simulink model "image_crop"  (R2016a)
settings: Solver=VariableStepAuto  StartTime=0.0  StopTime=1  RelTol=1e-3
libraries: visionsources x1
settings Model: Creator=Yewly  LastModifiedBy=Yewly

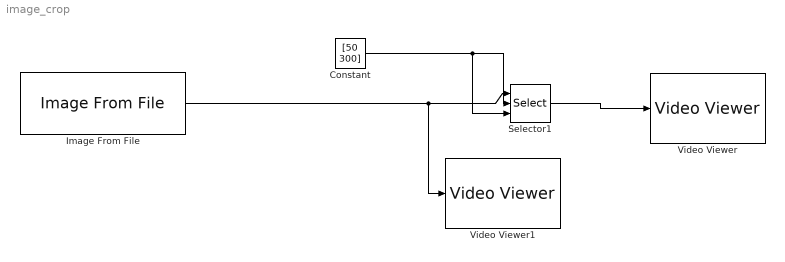
== system image_crop ==
  Constant : Constant  Value=[50 300]
  Image From File : visionsources/Image From File  Tag=vipblks_nd  FileName=color6.jpg  imagePorts=One multidimensional signal  Ts=1  ImageDataType=Inherit from input image  Signed=on  WordLength=16  sdImageDataType=uint(8)  FractionLengthMode=User-defined  FractionLength=15  OutPortLabels=R|G|B
  Selector1 : Selector  NumberOfDimensions=3  InputPortWidth=2  IndexOptions=Starting and ending indices (port),Starting and ending indices (port),Starting index (dialog)  Indices=50,50,1  OutputSizes=300,300,3
  Video Viewer : VideoViewer  FigPos=[886.6 726.8 540 585.6]
  Video Viewer1 : VideoViewer  FigPos=[285.8 732.4 540 585.6]
  wires:
  Selector1/1 -> Video Viewer/1
  Image From File/1 -> Selector1/1, Video Viewer1/1
  Constant/1 -> Selector1/3, Selector1/2
